simulink model "model1"  (Simulink 9.1)
settings: Solver=VariableStepDiscrete  StartTime=0.0  StopTime=20.0  RelTol=1e-3  EnableMultiTasking=on
settings Model: Creator=Admin  LastModifiedBy=Asus
settings DataIOCC: LimitDataPoints=on  SignalLoggingSaveFormat=ModelDataLogs
settings OptimizationCC: ExpressionDepthLimit=2147483647  InitFltsAndDblsToZero=on
settings DebuggingCC: SaveWithParameterizedLinksMsg=none  SignalResolutionControl=TryResolveAllWithWarning  SolverPrmCheckMsg=warning  MultiTaskDSMMsg=warning  MultiTaskCondExecSysMsg=none  FcnCallInpInsideContextMsg=warning  StateNameClashWarn=warning
settings GRTTargetCC: TargetFcnLib=ansi_tfl_tmw.mat  GeneratePreprocessorConditionals=Disable all

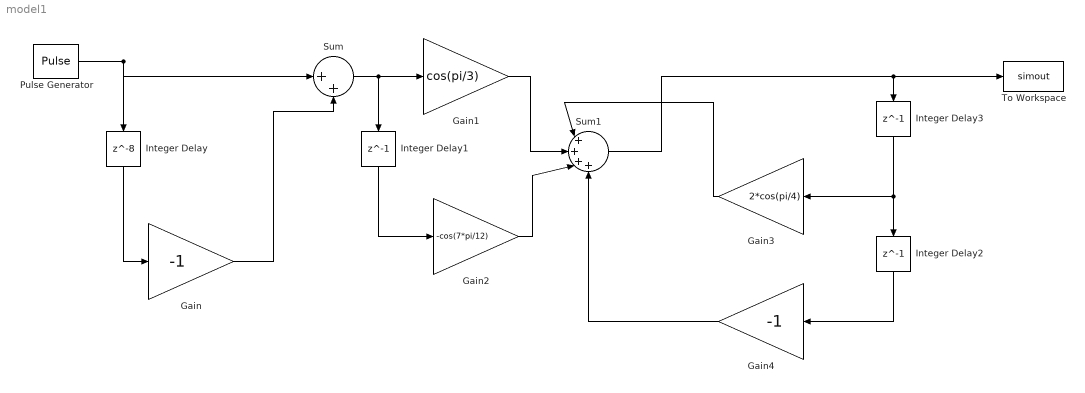
== system model1 ==
  Gain : Gain  Gain=-1
  Gain1 : Gain  Gain=cos(pi/3)
  Gain2 : Gain  Gain=-cos(7*pi/12)
  Gain3 : Gain  Gain=2*cos(pi/4)
  Gain4 : Gain  Gain=-1
  Integer Delay : Delay  DelayLength=8  InputProcessing=Inherited
  Integer Delay1 : Delay  DelayLength=1  InputProcessing=Inherited
  Integer Delay2 : Delay  DelayLength=1  InputProcessing=Inherited
  Integer Delay3 : Delay  DelayLength=1  InputProcessing=Inherited
  Pulse Generator : DiscretePulseGenerator  Period=100
  Sum : Sum  Inputs=|++
  Sum1 : Sum  Inputs=|++++
  To Workspace : ToWorkspace  VariableName=simout  SampleTime=-1
  wires:
  Integer Delay/1 -> Gain/1
  Sum/1 -> Gain1/1, Integer Delay1/1
  Pulse Generator/1 -> Integer Delay/1, Sum/1
  Gain/1 -> Sum/2
  Gain1/1 -> Sum1/2
  Integer Delay1/1 -> Gain2/1
  Gain2/1 -> Sum1/3
  Gain3/1 -> Sum1/1
  Gain4/1 -> Sum1/4
  Integer Delay2/1 -> Gain4/1
  Integer Delay3/1 -> Gain3/1, Integer Delay2/1
  Sum1/1 -> Integer Delay3/1, To Workspace/1
